simulink model "Decryption"  (R2022b)
settings: Solver=FixedStepAuto  StartTime=0.0  StopTime=10.0  RelTol=1e-3
settings Model: Creator=yuzehong  LastModifiedBy=sadamu
settings OptimizationCC: DefaultParameterBehavior=Inlined  UseDivisionForNetSlopeComputation=on  GainParamInheritBuiltInType=on  UseFloatMulNetSlope=on  InlineInvariantSignals=on  PassReuseOutputArgsAs=Individual arguments  NoFixptDivByZeroProtection=on  EfficientFloat2IntCast=on  LifeSpan=1  OptimizeBlockOrder=speed  DifferentSizesBufferReuse=on  EfficientTunableParamExpr=on
settings DebuggingCC: ParameterTunabilityLossMsg=error
settings HardwareCC: ProdLongLongMode=on
settings SFSimCC: MATLABDynamicMemAlloc=off
settings RTWCC: Description=Embedded Coder  SystemTargetFile=ert.tlc  GenCodeOnly=on  TemplateMakefile=ert_default_tmf
settings CodeAppCC: GenerateComments=off  IgnoreCustomStorageClasses=off  OperatorAnnotations=on  SimulinkDataObjDesc=on  SFDataObjDesc=on  CustomSymbolStrGlobalVar=rt$N$M  CustomSymbolStrType=$N$M  CustomSymbolStrFcn=$N$M$F  CustomSymbolStrMacro=$N$M  SimulinkBlockComments=off
settings ERTTargetCC: TargetLangStandard=C99 (ISO)  GenerateSampleERTMain=on  IncludeMdlTerminateFcn=off  CombineSignalStateStructs=on  SupportAbsoluteTime=off  CodeInterfacePackaging=Reusable function  SupportComplex=off  SupportContinuousTime=on  InlinedParameterPlacement=NonHierarchical  ERTCustomFileTemplate=example_file_process.tlc  ERTFilePackagingFormat=CompactWithDataFile

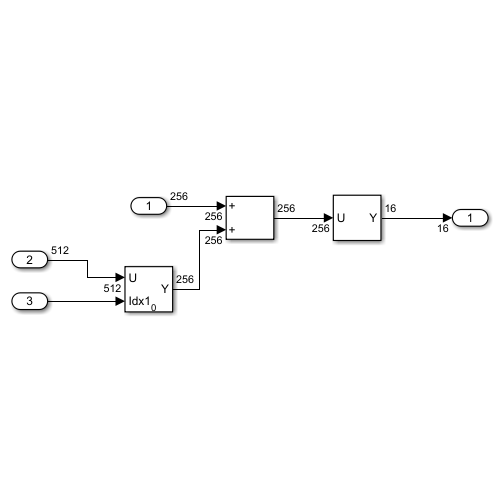
[thumbnail: Simulink's stored preview of the top-level diagram]
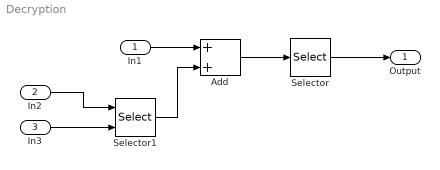
== system Decryption ==
  In1 : Inport  OutDataTypeStr=int32  PortDimensions=256
  In2 : Inport  Port=2  OutDataTypeStr=int32  PortDimensions=512
  In3 : Inport  Port=3  OutDataTypeStr=int32
  Add : Sum
  Selector : Selector  IndexMode=Zero-based  InputPortWidth=256  IndexOptions=Index vector (dialog)  Indices=[1 16 33 45 71 86 103 122 130 139 154 176 195 211 231 252]  OutputSizes=1
  Selector1 : Selector  IndexMode=Zero-based  InputPortWidth=512  IndexOptions=Starting index (port)  Indices=[1 3]  OutputSizes=256
  Output : Outport
  wires:
  Selector/1 -> Output/1
  In1/1 -> Add/1
  In2/1 -> Selector1/1
  Add/1 -> Selector/1
  Selector1/1 -> Add/2
  In3/1 -> Selector1/2
